simulink model "qr_array_cosim"  (R2017a)
settings: Solver=VariableStepAuto  StartTime=0.0  StopTime=600  RelTol=1e-3
values from neighbouring files (symbols this model uses):
  A = [0.69 0.5054 0.5914 0.5547 ... (first row only)    [load_data.m]
undefined symbols (not defined in the file or in its folder): N
libraries: xbsIndex_r4 x646, JTAGRuntimeCosim_r4 x1
(part 1 of 4)
settings Model: Creator=jhell  LastModifiedBy=jlh24

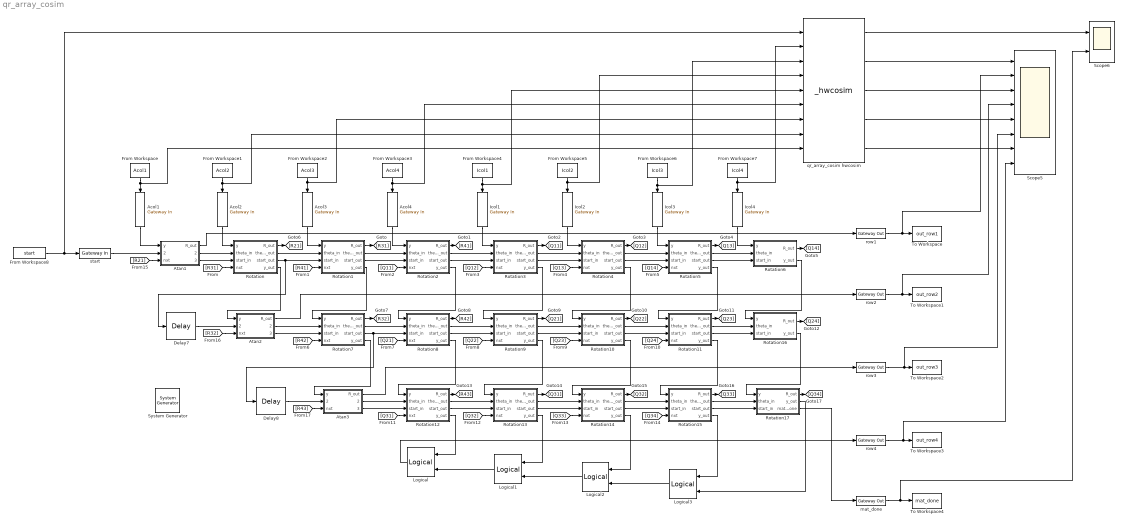
== system qr_array_cosim ==
  " System Generator" : xbsIndex_r4/ System Generator  Tag=genX  xilinxfamily=zynq  part=xc7z020  speed=-1  package=clg484  synthesis_tool=Vivado  clock_wrapper=Clock Enables  directory=./netlist_cosim  proj_type=Vivado  Synth_file=Vivado Synthesis Defaults  Impl_file=Vivado Implementation Defaults  testbench=off  simulink_period=1  sysclk_period=10  dcm_input_clock_period=10  incr_netlist=off  trim_vbits=Everywhere in SubSystem  dbl_ovrd=According to Block Masks  core_generation=According to Block Masks  run_coregen=off  deprecated_control=off  eval_field=0  block_type=sysgen
  Acol1 : xbsIndex_r4/Gateway In  gui_display_data_type=Fixed-point  arith_type="Signed  (2's comp)"  n_bits=16  bin_pt=13  preci_type=Single  exp_width=8  frac_width=24  rows=1  columns=1  quantization="Round  (unbiased: +/- Inf)"  overflow=Saturate  period=1  UseAsADC=off  ADCChannel='1'  interface=None  automatic_assignment=on  address_offset=hex2dec('00')  intf_name=''  intf_description=''  default_value=0  timing_constraint=None  locs_specified=off  LOCs={}  io_standard={}  inherit_from_input=off  hdl_port=on  dbl_ovrd=off  block_type=gatewayin
  Acol2 : xbsIndex_r4/Gateway In  gui_display_data_type=Fixed-point  arith_type="Signed  (2's comp)"  n_bits=16  bin_pt=13  preci_type=Single  exp_width=8  frac_width=24  rows=1  columns=1  quantization=Truncate  overflow=Saturate  period=1  UseAsADC=off  ADCChannel='1'  interface=None  automatic_assignment=on  address_offset=hex2dec('00')  intf_name=''  intf_description=''  default_value=0  timing_constraint=None  locs_specified=off  LOCs={}  io_standard={}  inherit_from_input=off  hdl_port=on  dbl_ovrd=off  block_type=gatewayin
  Acol3 : xbsIndex_r4/Gateway In  gui_display_data_type=Fixed-point  arith_type="Signed  (2's comp)"  n_bits=16  bin_pt=13  preci_type=Single  exp_width=8  frac_width=24  rows=1  columns=1  quantization=Truncate  overflow=Saturate  period=1  UseAsADC=off  ADCChannel='1'  interface=None  automatic_assignment=on  address_offset=hex2dec('00')  intf_name=''  intf_description=''  default_value=0  timing_constraint=None  locs_specified=off  LOCs={}  io_standard={}  inherit_from_input=off  hdl_port=on  dbl_ovrd=off  block_type=gatewayin
  Acol4 : xbsIndex_r4/Gateway In  gui_display_data_type=Fixed-point  arith_type="Signed  (2's comp)"  n_bits=16  bin_pt=13  preci_type=Single  exp_width=8  frac_width=24  rows=1  columns=1  quantization=Truncate  overflow=Saturate  period=1  UseAsADC=off  ADCChannel='1'  interface=None  automatic_assignment=on  address_offset=hex2dec('00')  intf_name=''  intf_description=''  default_value=0  timing_constraint=None  locs_specified=off  LOCs={}  io_standard={}  inherit_from_input=off  hdl_port=on  dbl_ovrd=off  block_type=gatewayin
  Atan1 : Subsystem
  Atan2 : Subsystem
  Atan3 : Subsystem
  Delay7 : xbsIndex_r4/Delay  rst=off  infoeditControl=Selection of Reset will increase slice count due to use of real FFs and instead of SRLs  en=off  latency=43  reg_retiming=off  dbl_ovrd=off  block_type=delay
  Delay8 : xbsIndex_r4/Delay  rst=off  infoeditControl=Selection of Reset will increase slice count due to use of real FFs and instead of SRLs  en=off  latency=43  reg_retiming=off  dbl_ovrd=off  block_type=delay
  From Workspace : FromWorkspace  VariableName=Acol1  SampleTime=0  Interpolate=off  OutputAfterFinalValue=Setting to zero
  From Workspace1 : FromWorkspace  VariableName=Acol2  SampleTime=0  Interpolate=off  OutputAfterFinalValue=Setting to zero
  From Workspace2 : FromWorkspace  VariableName=Acol3  SampleTime=0  Interpolate=off  OutputAfterFinalValue=Setting to zero
  From Workspace3 : FromWorkspace  VariableName=Acol4  SampleTime=0  Interpolate=off  OutputAfterFinalValue=Setting to zero
  From Workspace4 : FromWorkspace  VariableName=Icol1  SampleTime=0  Interpolate=off  OutputAfterFinalValue=Setting to zero
  From Workspace5 : FromWorkspace  VariableName=Icol2  SampleTime=0  Interpolate=off  OutputAfterFinalValue=Setting to zero
  From Workspace6 : FromWorkspace  VariableName=Icol3  SampleTime=0  Interpolate=off  OutputAfterFinalValue=Setting to zero
  From Workspace7 : FromWorkspace  VariableName=Icol4  SampleTime=0  Interpolate=off  OutputAfterFinalValue=Setting to zero
  From Workspace8 : FromWorkspace  VariableName=start  SampleTime=0
  Icol{1..4} (4 alike) : xbsIndex_r4/Gateway In  gui_display_data_type=Fixed-point  arith_type="Signed  (2's comp)"  n_bits=16  bin_pt=13  preci_type=Single  exp_width=8  frac_width=24  rows=1  columns=1  quantization=Truncate  overflow=Saturate  period=1  UseAsADC=off  ADCChannel='1'  interface=None  automatic_assignment=on  address_offset=hex2dec('00')  intf_name=''  intf_description=''  default_value=0  timing_constraint=None  locs_specified=off  LOCs={}  io_standard={}  inherit_from_input=off  hdl_port=on  dbl_ovrd=off  block_type=gatewayin
  Logical{,1..3} (4 alike) : xbsIndex_r4/Logical  logical_function=OR  inputs=2  en=off  latency=1  precision=Full  arith_type=Unsigned  n_bits=16  bin_pt=0  align_bp=on  dbl_ovrd=off  block_type=logical
  Rotation : Subsystem
  Rotation1 : Subsystem
  Rotation10 : Subsystem
  Rotation11 : Subsystem
  Rotation12 : Subsystem
  Rotation13 : Subsystem
  Rotation14 : Subsystem
  Rotation15 : Subsystem
  Rotation16 : Subsystem
  Rotation17 : Subsystem
  Rotation2 : Subsystem
  Rotation3 : Subsystem
  Rotation4 : Subsystem
  Rotation5 : Subsystem
  Rotation6 : Subsystem
  Rotation7 : Subsystem
  Rotation8 : Subsystem
  Rotation9 : Subsystem
  Scope5 : Scope  NumInputPorts=8
  Scope6 : Scope  NumInputPorts=2
  To Workspace : ToWorkspace  VariableName=out_row1  SampleTime=-1
  To Workspace1 : ToWorkspace  VariableName=out_row2  SampleTime=-1
  To Workspace2 : ToWorkspace  VariableName=out_row3  SampleTime=-1
  To Workspace3 : ToWorkspace  VariableName=out_row4  SampleTime=-1
  To Workspace4 : ToWorkspace  VariableName=mat_done  SampleTime=-1
  mat_done : xbsIndex_r4/Gateway Out  inherit_from_input=off  hdl_port=on  rows=1  columns=1  UseAsDAC=off  DACChannel='1'  interface=None  automatic_assignment=on  address_offset=hex2dec('00')  intf_name=''  intf_description=''  timing_constraint=None  locs_specified=off  LOCs={}  io_standard={}  block_type=gatewayout
  qr_array_cosim hwcosim : JTAGRuntimeCosim_r4/_hwcosim  clkSrc=Single Stepped  hasCombinationalPath=on  bitfileName=C:\ELEC522\hellar\Project_5\netlist_cosim\qr_array_cosim.bit  skipConfig=off  dispPartInfo=off  useZynqReconfigScript=on  cable=Auto Detect  speed=N/A  cablePort=N/A  cableLocation=Local  shareCable=off  design_xtable=|  engineDll=JTAGCosimEngine.dll  cableWaitTime=10  bscanPos=-1  IRLengths=[]  useWaitBox=1  hasBufgmux=on  Scheme=Cosim  useCmdProc=1  hasProc=0  useImpact=0  printLogFile=0  userChain=2  block_type=jtagcosim
      | {
      |     'clkWrapper' => 'qr_array_cosim',
      |     'burstMode' => false,
      |     'burstFifoDepth' => '1024',
      |     'shared_memories' => {},
      |     'clocksGcd' => 1,
      |     'device' => {
      |       'family' => 'zynq',
      |       'part' => 'xc7z020',
      |       'package' => 'clg484',
      |       'speed' => '-1',
      |     },
      |     'ports' => {
      |       'start' => {
      |         'direction' => 'in',
      |         'width' => 1,
      |         'name' => 'start',
      |         'period' => 1,
      |         'icon_text' => 'start',
      |         'type' => 'Bool',
      |         'arithmetic_type' => 'xlUnsigned',
      |         'dat_file' => 'qr_array_cosim_start.dat',
      |         'bin_pt' => 0,
      |         'addr_offset' => 0,
      |         'bd_port_index' => 0,
      |       },
      |       'icol4' => {
      |         'direction' => 'in',
      |         'width' => 16,
      |         'name' => 'icol4',
      |         'period' => 1,
      |         'icon_text' => 'Icol4',
      |         'type' => 'Fix_16_13',
      |         'arithmetic_type' => 'xlSigned',
      |         'dat_file' => 'qr_array_cosim_icol4.dat',
      |         'bin_pt' => 13,
      |         'addr_offset' => 4,
      |         'bd_port_index' => 1,
      |       },
      |       'icol3' => {
      |         'direction' => 'in',
      |         'width' => 16,
      |         'name' => 'icol3',
      |         'period' => 1,
      |         'icon_text' => 'Icol3',
      |         'type' => 'Fix_16_13',
      |         'arithmetic_type' => 'xlSigned',
      |         'dat_file' => 'qr_array_cosim_icol3.dat',
      |         'bin_pt' => 13,
      |         'addr_offset' => 8,
      |         'bd_port_index' => 2,
      |       },
      |       'icol2' => {
      |         'direction' => 'in',
      |         'width' => 16,
      |         'name' => 'icol2',
      |         'period' => 1,
      |         'icon_text' => 'Icol2',
      |         'type' => 'Fix_16_13',
      |         'arithmetic_type' => 'xlSigned',
      |         'dat_file' => 'qr_array_cosim_icol2.dat',
      |         'bin_pt' => 13,
      |         'addr_offset' => 12,
      |         'bd_port_index' => 3,
      |       },
      |       'icol1' => {
      |         'direction' => 'in',
      |         'width' => 16,
      |         'name' => 'icol1',
      |         'period' => 1,
      |         'icon_text' => 'Icol1',
      |         'type' => 'Fix_16_13',
      |         'arithmetic_type' => 'xlSigned',
      |         'dat_file' => 'qr_array_cosim_icol1.dat',
      |         'bin_pt' => 13,
      |         'addr_offset' => 16,
      |         'bd_port_index' => 4,
      |       },
      |       'acol4' => {
      |         'direction' => 'in',
      |         'width' => 16,
      |         'name' => 'acol4',
      |         'period' => 1,
      |         'icon_text' => 'Acol4',
      |         'type' => 'Fix_16_13',
      |         'arithmetic_type' => 'xlSigned',
      |         'dat_file' => 'qr_array_cosim_acol4.dat',
      |         'bin_pt' => 13,
      |         'addr_offset' => 20,
      |         'bd_port_index' => 5,
      |       },
      |       'acol3' => {
      |         'direction' => 'in',
      |         'width' => 16,
      |         'name' => 'acol3',
      |         'period' => 1,
      |         'icon_text' => 'Acol3',
      |         'type' => 'Fix_16_13',
      |         'arithmetic_type' => 'xlSigned',
      |         'dat_file' => 'qr_array_cosim_acol3.dat',
      |         'bin_pt' => 13,
      |         'addr_offset' => 24,
      |         'bd_port_index' => 6,
      |       },
      |       'acol2' => {
      |         'direction' => 'in',
      |         'width' => 16,
      |         'name' => 'acol2',
      |         'period' => 1,
      |         'icon_text' => 'Acol2',
      |         'type' => 'Fix_16_13',
      |         'arithmetic_type' => 'xlSigned',
      |         'dat_file' => 'qr_array_cosim_acol2.dat',
      |         'bin_pt' => 13,
      |         'addr_offset' => 28,
      |         'bd_port_index' => 7,
      |       },
      |       'acol1' => {
      |         'direction' => 'in',
      |         'width' => 16,
      |         'name' => 'acol1',
      |         'period' => 1,
      |         'icon_text' => 'Acol1',
      |         'type' => 'Fix_16_13',
      |         'arithmetic_type' => 'xlSigned',
      |         'dat_file' => 'qr_array_cosim_acol1.dat',
      |         'bin_pt' => 13,
      |         'addr_offset' => 32,
      |         'bd_port_index' => 8,
      |       },
      |       'mat_done' => {
      |         'direction' => 'out',
      |         'width' => 1,
      |         'name' => 'mat_done',
      |         'period' => 1,
      |         'icon_text' => 'mat_done',
      |         'type' => 'Bool',
      |         'arithmetic_type' => 'xlUnsigned',
      |         'dat_file' => 'qr_array_cosim_mat_done.dat',
      |         'bin_pt' => 0,
      |         'addr_offset' => 36,
      |         'bd_port_index' => 0,
      |       },
      |       'row1' => {
      |         'direction' => 'out',
      |         'width' => 16,
      |         'name' => 'row1',
      |         'period' => 1,
      |         'icon_text' => 'row1',
      |         'type' => 'Fix_16_13',
      |         'arithmetic_type' => 'xlSigned',
      |         'dat_file' => 'qr_array_cosim_row1.dat',
      |         'bin_pt' => 13,
      |         'addr_offset' => 40,
      |         'bd_port_index' => 1,
      |       },
      |       'row2' => {
      |         'direction' => 'out',
      |         'width' => 16,
      |         'name' => 'row2',
      |         'period' => 1,
      |         'icon_text' => 'row2',
      |         'type' => 'Fix_16_13',
      |         'arithmetic_type' => 'xlSigned',
      |         'dat_file' => 'qr_array_cosim_row2.dat',
      |         'bin_pt' => 13,
      |         'addr_offset' => 44,
      |         'bd_port_index' => 2,
      |       },
      |       'row3' => {
      |         'direction' => 'out',
      |         'width' => 16,
      |         'name' => 'row3',
      |         'period' => 1,
      |         'icon_text' => 'row3',
      |         'type' => 'Fix_16_13',
      |         'arithmetic_type' => 'xlSigned',
      |         'dat_file' => 'qr_array_cosim_row3.dat',
      |         'bin_pt' => 13,
      |         'addr_offset' => 48,
      |         'bd_port_index' => 3,
      |       },
      |       'row4' => {
      |         'direction' => 'out',
      |         'width' => 16,
      |         'name' => 'row4',
      |         'period' => 1,
      |         'icon_text' => 'row4',
      |         'type' => 'Fix_16_13',
      |         'arithmetic_type' => 'xlSigned',
      |         'dat_file' => 'qr_array_cosim_row4.dat',
      |         'bin_pt' => 13,
      |         'addr_offset' => 52,
      |         'bd_port_index' => 4,
      |       },
      |     },
      |   }
  row{1..4} (4 alike) : xbsIndex_r4/Gateway Out  inherit_from_input=off  hdl_port=on  rows=1  columns=1  UseAsDAC=off  DACChannel='1'  interface=None  automatic_assignment=on  address_offset=hex2dec('00')  intf_name=''  intf_description=''  timing_constraint=None  locs_specified=off  LOCs={}  io_standard={}  block_type=gatewayout
  start : xbsIndex_r4/Gateway In  gui_display_data_type=Boolean  arith_type=Boolean  n_bits=16  bin_pt=14  preci_type=Single  exp_width=8  frac_width=24  rows=1  columns=1  quantization="Round  (unbiased: +/- Inf)"  overflow=Saturate  period=1  UseAsADC=off  ADCChannel='1'  interface=None  automatic_assignment=on  address_offset=hex2dec('00')  intf_name=''  intf_description=''  default_value=0  timing_constraint=None  locs_specified=off  LOCs={}  io_standard={}  inherit_from_input=off  hdl_port=on  dbl_ovrd=off  block_type=gatewayin
  wires:
  From Workspace2/1 -> qr_array_cosim hwcosim/7, Acol3/1
  From Workspace3/1 -> qr_array_cosim hwcosim/6, Acol4/1
  From Workspace/1 -> qr_array_cosim hwcosim/9, Acol1/1
  From Workspace4/1 -> qr_array_cosim hwcosim/5, Icol1/1
  From Workspace5/1 -> qr_array_cosim hwcosim/4, Icol2/1
  From Workspace6/1 -> qr_array_cosim hwcosim/3, Icol3/1
  From Workspace7/1 -> qr_array_cosim hwcosim/2, Icol4/1
  Rotation/2(theta_out) -> Rotation1/2(theta_in)
  Rotation/3(start_out) -> Rotation1/3(start_in), Delay7/1
  Rotation1/2(theta_out) -> Rotation2/2(theta_in)
  Rotation1/3(start_out) -> Rotation2/3(start_in)
  Rotation2/2(theta_out) -> Rotation3/2(theta_in)
  Rotation2/3(start_out) -> Rotation3/3(start_in)
  Rotation3/2(theta_out) -> Rotation4/2(theta_in)
  Rotation3/3(start_out) -> Rotation4/3(start_in)
  Rotation4/2(theta_out) -> Rotation5/2(theta_in)
  Rotation4/3(start_out) -> Rotation5/3(start_in)
  Rotation5/2(theta_out) -> Rotation6/2(theta_in)
  Rotation5/3(start_out) -> Rotation6/3(start_in)
  Rotation1/1(R_out) -> [R31]
  [R31] -> Rotation/4(nxt)
  Rotation2/1(R_out) -> [R41]
  [R41] -> Rotation1/4(nxt)
  Rotation3/1(R_out) -> [Q11]
  Rotation4/1(R_out) -> [Q12]
  Rotation5/1(R_out) -> [Q13]
  Rotation6/1(R_out) -> [Q14]
  [Q11] -> Rotation2/4(nxt)
  [Q12] -> Rotation3/4(nxt)
  [Q13] -> Rotation4/4(nxt)
  [Q14] -> Rotation5/4(nxt)
  row1/1 -> Scope5/2, To Workspace/1
  Rotation7/2(theta_out) -> Rotation8/2(theta_in)
  Rotation7/3(start_out) -> Rotation8/3(start_in), Delay8/1
  Rotation8/2(theta_out) -> Rotation9/2(theta_in)
  Rotation8/3(start_out) -> Rotation9/3(start_in)
  Rotation9/2(theta_out) -> Rotation10/2(theta_in)
  Rotation9/3(start_out) -> Rotation10/3(start_in)
  Rotation10/2(theta_out) -> Rotation11/2(theta_in)
  Rotation10/3(start_out) -> Rotation11/3(start_in)
  Rotation1/4(y_out) -> Rotation7/1(y)
  Rotation2/4(y_out) -> Rotation8/1(y)
  Rotation3/4(y_out) -> Rotation9/1(y)
  Rotation4/4(y_out) -> Rotation10/1(y)
  Rotation5/4(y_out) -> Rotation11/1(y)
  Rotation11/3(start_out) -> Rotation16/3(start_in)
  Rotation11/2(theta_out) -> Rotation16/2(theta_in)
  Rotation6/2(y_out) -> Rotation16/1(y)
  Rotation16/2(y_out) -> Rotation17/1(y)
  Rotation/1(R_out) -> [R21]
  Rotation8/1(R_out) -> [R42]
  Rotation9/1(R_out) -> [Q21]
  Rotation10/1(R_out) -> [Q22]
  Rotation11/1(R_out) -> [Q23]
  Rotation16/1(R_out) -> [Q24]
  [R42] -> Rotation7/4(nxt)
  [Q21] -> Rotation8/4(nxt)
  [Q22] -> Rotation9/4(nxt)
  [Q23] -> Rotation10/4(nxt)
  [Q24] -> Rotation11/4(nxt)
  Rotation8/4(y_out) -> Rotation12/1(y)
  Rotation12/2(theta_out) -> Rotation13/2(theta_in)
  Rotation12/3(start_out) -> Rotation13/3(start_in)
  Rotation13/2(theta_out) -> Rotation14/2(theta_in)
  Rotation13/3(start_out) -> Rotation14/3(start_in)
  Rotation14/2(theta_out) -> Rotation15/2(theta_in)
  Rotation14/3(start_out) -> Rotation15/3(start_in)
  Rotation15/2(theta_out) -> Rotation17/2(theta_in)
  Rotation9/4(y_out) -> Rotation13/1(y)
  Rotation10/4(y_out) -> Rotation14/1(y)
  Rotation11/4(y_out) -> Rotation15/1(y)
  Rotation12/1(R_out) -> [R43]
  Rotation13/1(R_out) -> [Q31]
  Rotation14/1(R_out) -> [Q32]
  Rotation15/1(R_out) -> [Q33]
  Rotation17/1(R_out) -> [Q34]
  Rotation15/3(start_out) -> Rotation17/3(start_in)
  [Q31] -> Rotation12/4(nxt)
  [Q32] -> Rotation13/4(nxt)
  [Q33] -> Rotation14/4(nxt)
  [Q34] -> Rotation15/4(nxt)
  row2/1 -> Scope5/4, To Workspace1/1
  row3/1 -> Scope5/6, To Workspace2/1
  row4/1 -> Scope5/8, To Workspace3/1
  Atan1/2(theta_out) -> Rotation/2(theta_in)
  Atan1/3(start_out) -> Rotation/3(start_in)
  Atan1/1(R_out) -> row1/1
  [R21] -> Atan1/3(nxt)
  Acol1/1 -> Atan1/1(y)
  Atan2/2(theta_out) -> Rotation7/2(theta_in)
  Atan2/3(start_out) -> Rotation7/3(start_in)
  Atan2/1(R_out) -> row2/1
  Rotation/4(y_out) -> Atan2/1(y)
  [R32] -> Atan2/3(nxt)
  Atan3/3(start_out) -> Rotation12/3(start_in)
  Rotation7/4(y_out) -> Atan3/1(y)
  Atan3/1(R_out) -> row3/1
  From Workspace8/1 -> qr_array_cosim hwcosim/1, start/1
  start/1 -> Atan1/2(start_in)
  Acol2/1 -> Rotation/1(y)
  Acol3/1 -> Rotation1/1(y)
  Acol4/1 -> Rotation2/1(y)
  Icol1/1 -> Rotation3/1(y)
  Icol2/1 -> Rotation4/1(y)
  Icol3/1 -> Rotation5/1(y)
  Icol4/1 -> Rotation6/1(y)
  [R43] -> Atan3/3(nxt)
  Delay7/1 -> Atan2/2(start_in)
  Delay8/1 -> Atan3/2(start_in)
  Rotation7/1(R_out) -> [R32]
  Atan3/2(theta_out) -> Rotation12/2(theta_in)
  Rotation17/3(mat_done) -> mat_done/1
  mat_done/1 -> Scope6/2, To Workspace4/1
  Rotation12/4(y_out) -> Logical/1
  Logical1/1 -> Logical/2
  Rotation13/4(y_out) -> Logical1/1
  Rotation14/4(y_out) -> Logical2/1
  Logical2/1 -> Logical1/2
  Logical3/1 -> Logical2/2
  Rotation15/4(y_out) -> Logical3/1
  Rotation17/2(y_out) -> Logical3/2
  Logical/1 -> row4/1
  From Workspace1/1 -> qr_array_cosim hwcosim/8, Acol2/1
  qr_array_cosim hwcosim/2 -> Scope5/1
  qr_array_cosim hwcosim/3 -> Scope5/3
  qr_array_cosim hwcosim/4 -> Scope5/5
  qr_array_cosim hwcosim/5 -> Scope5/7
  qr_array_cosim hwcosim/1 -> Scope6/1

== system qr_array_cosim/Atan1 ==
  note: GenerateCordicEnable
  note: GenerateQRDone
  y : Inport
  start_in : Inport  Port=2
  nxt : Inport  Port=3
  Accumulator : xbsIndex_r4/Accumulator  operation=Add  n_bits=8  overflow=Wrap  scale=1  rst=on  hasbypass=off  infoeditControl=reset for floating point data type must be asserted for a minimum of 2 cycles  en=on  latency=1  msb_inp=100  msb=100  lsb=-100  use_behavioral_HDL=on  implementation=Fabric  dbl_ovrd=off  block_type=accum
  Constant : xbsIndex_r4/Constant  const=0  gui_display_data_type=Fixed-point  arith_type=Signed (2's comp)  n_bits=16  bin_pt=13  preci_type=Single  exp_width=8  frac_width=24  explicit_period=off  period=1  equ=P=C  opselect=C  inp2=PCIN>>17  opr=+  inp1=P  carry=CIN  dbl_ovrd=off  block_type=constant
  Constant1 : xbsIndex_r4/Constant  const=1  gui_display_data_type=Fixed-point  arith_type=Unsigned  n_bits=16  bin_pt=0  preci_type=Single  exp_width=8  frac_width=24  explicit_period=off  period=1  equ=P=C  opselect=C  inp2=PCIN>>17  opr=+  inp1=P  carry=CIN  dbl_ovrd=off  block_type=constant
  Constant2 : xbsIndex_r4/Constant  const=0  gui_display_data_type=Boolean  arith_type=Boolean  n_bits=16  bin_pt=14  preci_type=Single  exp_width=8  frac_width=24  explicit_period=off  period=1  equ=P=C  opselect=C  inp2=PCIN>>17  opr=+  inp1=P  carry=CIN  dbl_ovrd=off  block_type=constant
  Constant4 : xbsIndex_r4/Constant  const=0  gui_display_data_type=Fixed-point  arith_type=Signed (2's comp)  n_bits=16  bin_pt=13  preci_type=Single  exp_width=8  frac_width=24  explicit_period=off  period=1  equ=P=C  opselect=C  inp2=PCIN>>17  opr=+  inp1=P  carry=CIN  dbl_ovrd=off  block_type=constant
  Constant5 : xbsIndex_r4/Constant  const=0  gui_display_data_type=Fixed-point  arith_type=Unsigned  n_bits=16  bin_pt=0  preci_type=Single  exp_width=8  frac_width=24  explicit_period=off  period=1  equ=P=C  opselect=C  inp2=PCIN>>17  opr=+  inp1=P  carry=CIN  dbl_ovrd=off  block_type=constant
  Constant6 : xbsIndex_r4/Constant  const=4  gui_display_data_type=Fixed-point  arith_type=Unsigned  n_bits=16  bin_pt=0  preci_type=Single  exp_width=8  frac_width=24  explicit_period=off  period=1  equ=P=C  opselect=C  inp2=PCIN>>17  opr=+  inp1=P  carry=CIN  dbl_ovrd=off  block_type=constant
  Delay : xbsIndex_r4/Delay  rst=off  infoeditControl=Selection of Reset will increase slice count due to use of real FFs and instead of SRLs  en=off  latency=1  reg_retiming=off  dbl_ovrd=off  block_type=delay
  Delay4 : xbsIndex_r4/Delay  rst=off  infoeditControl=Selection of Reset will increase slice count due to use of real FFs and instead of SRLs  en=off  latency=4  reg_retiming=off  dbl_ovrd=off  block_type=delay
  Delay5 : xbsIndex_r4/Delay  rst=off  infoeditControl=Selection of Reset will increase slice count due to use of real FFs and instead of SRLs  en=off  latency=1  reg_retiming=off  dbl_ovrd=off  block_type=delay
  Delay6 : xbsIndex_r4/Delay  rst=off  infoeditControl=Selection of Reset will increase slice count due to use of real FFs and instead of SRLs  en=off  latency=44  reg_retiming=off  dbl_ovrd=off  block_type=delay
  Delay7 : xbsIndex_r4/Delay  rst=off  infoeditControl=Selection of Reset will increase slice count due to use of real FFs and instead of SRLs  en=off  latency=43  reg_retiming=off  dbl_ovrd=off  block_type=delay
  Delay8 : xbsIndex_r4/Delay  rst=off  infoeditControl=Selection of Reset will increase slice count due to use of real FFs and instead of SRLs  en=off  latency=2  reg_retiming=off  dbl_ovrd=off  block_type=delay
  Inverter : xbsIndex_r4/Inverter  en=off  latency=1  dbl_ovrd=off  block_type=inv
  Logical : xbsIndex_r4/Logical  logical_function=OR  inputs=2  en=off  latency=1  precision=Full  arith_type=Unsigned  n_bits=16  bin_pt=0  align_bp=on  dbl_ovrd=off  block_type=logical
  Logical3 : xbsIndex_r4/Logical  logical_function=XOR  inputs=2  en=off  latency=0  precision=Full  arith_type=Unsigned  n_bits=16  bin_pt=0  align_bp=on  dbl_ovrd=off  block_type=logical
  Logical4 : xbsIndex_r4/Logical  logical_function=OR  inputs=2  en=off  latency=1  precision=Full  arith_type=Unsigned  n_bits=16  bin_pt=0  align_bp=on  dbl_ovrd=off  block_type=logical
  Logical5 : xbsIndex_r4/Logical  logical_function=OR  inputs=2  en=off  latency=0  precision=Full  arith_type=Unsigned  n_bits=16  bin_pt=0  align_bp=on  dbl_ovrd=off  block_type=logical
  Logical6 : xbsIndex_r4/Logical  logical_function=XOR  inputs=2  en=off  latency=1  precision=Full  arith_type=Unsigned  n_bits=16  bin_pt=0  align_bp=on  dbl_ovrd=off  block_type=logical
  Logical7 : xbsIndex_r4/Logical  logical_function=OR  inputs=2  en=off  latency=1  precision=Full  arith_type=Unsigned  n_bits=16  bin_pt=0  align_bp=on  dbl_ovrd=off  block_type=logical
  Logical8 : xbsIndex_r4/Logical  logical_function=AND  inputs=2  en=off  latency=1  precision=Full  arith_type=Unsigned  n_bits=16  bin_pt=0  align_bp=on  dbl_ovrd=off  block_type=logical
  Mux{,1..3} (4 alike) : xbsIndex_r4/Mux  inputs=2  en=off  latency=1  precision=Full  arith_type=Unsigned  n_bits=16  bin_pt=14  quantization=Truncate  overflow=Wrap  dbl_ovrd=off  block_type=mux
  Register : xbsIndex_r4/Register  init=0  rst=on  en=on  dbl_ovrd=off  block_type=register
  Register2 : xbsIndex_r4/Register  init=0  rst=off  en=on  dbl_ovrd=off  block_type=register
  Relational : xbsIndex_r4/Relational  mode=a=b  op_type=Bool  en=off  latency=0  dbl_ovrd=off  block_type=relational
  Terminator{1..5} (5 alike) : Terminator
  Vivado HLS : xbsIndex_r4/Vivado HLS  anytable='C:/ELEC522/hellar/Project_4/cordic_revised/cordic_revised/solution1'  fast_sim=off  display_datatype=on  rate_propagation_method=Simulink system period  model_file_path=''  latency=1  block_type=hls
      settings: infoedit=This block allows including C,C++ and SystemC source files in System Generator for DSP designs.
  R_out : Outport
  theta_out : Outport  Port=2
  start_out : Outport  Port=3
  wires:
  Delay4/1 -> Vivado HLS/1
  Vivado HLS/2 -> Terminator2/1
  Constant4/1 -> Mux1/3
  Constant2/1 -> Vivado HLS/3
  Mux/1 -> Register/1
  Vivado HLS/1 -> Terminator4/1
  Constant/1 -> Vivado HLS/6
  y/1 -> Mux/3, Vivado HLS/4
  Vivado HLS/5 -> [R_vld]
  [R_out] -> Mux/2
  nxt/1 -> Mux2/2
  Vivado HLS/3 -> Terminator3/1
  Vivado HLS/6 -> Terminator5/1
  Vivado HLS/7 -> Terminator1/1
  Vivado HLS/8 -> Register2/1
  Vivado HLS/9 -> Register2/2
  start_in/1 -> [new_mat], Delay6/1
  Vivado HLS/4 -> [R_out]
  [done] -> Delay/1
  Delay/1 -> Register/2
  [R_vld] -> Delay8/1, Logical/2
  [reg_internal] -> Mux1/2
  Register/1 -> Mux2/3, [reg_internal]
  [done] -> Delay4/1
  [new_mat] -> Mux1/1
  [new_mat] -> Mux/1
  [new_mat] -> Logical/1
  [done] -> Mux2/1
  Logical/1 -> Register/3
  Delay8/1 -> [data_ready]
  Logical8/1 -> Vivado HLS/2, [enable]
  Register2/1 -> Inverter/1
  Delay6/1 -> start_out/1
  Mux2/1 -> R_out/1
  Relational/1 -> Logical4/2, Accumulator/2, [done]
  Mux1/1 -> Vivado HLS/5
  Inverter/1 -> theta_out/1
  Delay5/1 -> Logical3/1, Accumulator/3
  Logical3/1 -> Delay5/1
  Logical4/1 -> Logical3/2
  [new_mat] -> Logical4/1
  Constant6/1 -> Relational/2
  Constant5/1 -> Mux3/2
  Constant1/1 -> Mux3/3
  Accumulator/1 -> Relational/1
  Mux3/1 -> Accumulator/1
  [enable] -> Mux3/1
  Logical5/1 -> Logical8/1
  Logical7/1 -> Logical6/2
  Logical6/1 -> Logical6/1, Logical8/2
  [done] -> Logical7/2
  [new_mat] -> Delay7/1, Logical7/1
  Delay7/1 -> Logical5/2
  [data_ready] -> Logical5/1

== system qr_array_cosim/Atan2 ==
  note: GenerateCordicEnable
  note: GenerateQRDone
  y : Inport
  start_in : Inport  Port=2
  nxt : Inport  Port=3
  Accumulator : xbsIndex_r4/Accumulator  operation=Add  n_bits=8  overflow=Wrap  scale=1  rst=on  hasbypass=off  infoeditControl=reset for floating point data type must be asserted for a minimum of 2 cycles  en=on  latency=1  msb_inp=100  msb=100  lsb=-100  use_behavioral_HDL=on  implementation=Fabric  dbl_ovrd=off  block_type=accum
  Constant : xbsIndex_r4/Constant  const=0  gui_display_data_type=Fixed-point  arith_type=Signed (2's comp)  n_bits=16  bin_pt=13  preci_type=Single  exp_width=8  frac_width=24  explicit_period=off  period=1  equ=P=C  opselect=C  inp2=PCIN>>17  opr=+  inp1=P  carry=CIN  dbl_ovrd=off  block_type=constant
  Constant1 : xbsIndex_r4/Constant  const=1  gui_display_data_type=Fixed-point  arith_type=Unsigned  n_bits=16  bin_pt=0  preci_type=Single  exp_width=8  frac_width=24  explicit_period=off  period=1  equ=P=C  opselect=C  inp2=PCIN>>17  opr=+  inp1=P  carry=CIN  dbl_ovrd=off  block_type=constant
  Constant2 : xbsIndex_r4/Constant  const=0  gui_display_data_type=Boolean  arith_type=Boolean  n_bits=16  bin_pt=14  preci_type=Single  exp_width=8  frac_width=24  explicit_period=off  period=1  equ=P=C  opselect=C  inp2=PCIN>>17  opr=+  inp1=P  carry=CIN  dbl_ovrd=off  block_type=constant
  Constant4 : xbsIndex_r4/Constant  const=0  gui_display_data_type=Fixed-point  arith_type=Signed (2's comp)  n_bits=16  bin_pt=13  preci_type=Single  exp_width=8  frac_width=24  explicit_period=off  period=1  equ=P=C  opselect=C  inp2=PCIN>>17  opr=+  inp1=P  carry=CIN  dbl_ovrd=off  block_type=constant
  Constant5 : xbsIndex_r4/Constant  const=0  gui_display_data_type=Fixed-point  arith_type=Unsigned  n_bits=16  bin_pt=0  preci_type=Single  exp_width=8  frac_width=24  explicit_period=off  period=1  equ=P=C  opselect=C  inp2=PCIN>>17  opr=+  inp1=P  carry=CIN  dbl_ovrd=off  block_type=constant
  Constant6 : xbsIndex_r4/Constant  const=3  gui_display_data_type=Fixed-point  arith_type=Unsigned  n_bits=16  bin_pt=0  preci_type=Single  exp_width=8  frac_width=24  explicit_period=off  period=1  equ=P=C  opselect=C  inp2=PCIN>>17  opr=+  inp1=P  carry=CIN  dbl_ovrd=off  block_type=constant
  Delay : xbsIndex_r4/Delay  rst=off  infoeditControl=Selection of Reset will increase slice count due to use of real FFs and instead of SRLs  en=off  latency=1  reg_retiming=off  dbl_ovrd=off  block_type=delay
  Delay4 : xbsIndex_r4/Delay  rst=off  infoeditControl=Selection of Reset will increase slice count due to use of real FFs and instead of SRLs  en=off  latency=4  reg_retiming=off  dbl_ovrd=off  block_type=delay
  Delay5 : xbsIndex_r4/Delay  rst=off  infoeditControl=Selection of Reset will increase slice count due to use of real FFs and instead of SRLs  en=off  latency=1  reg_retiming=off  dbl_ovrd=off  block_type=delay
  Delay6 : xbsIndex_r4/Delay  rst=off  infoeditControl=Selection of Reset will increase slice count due to use of real FFs and instead of SRLs  en=off  latency=44  reg_retiming=off  dbl_ovrd=off  block_type=delay
  Delay7 : xbsIndex_r4/Delay  rst=off  infoeditControl=Selection of Reset will increase slice count due to use of real FFs and instead of SRLs  en=off  latency=43  reg_retiming=off  dbl_ovrd=off  block_type=delay
  Delay8 : xbsIndex_r4/Delay  rst=off  infoeditControl=Selection of Reset will increase slice count due to use of real FFs and instead of SRLs  en=off  latency=2  reg_retiming=off  dbl_ovrd=off  block_type=delay
  Inverter : xbsIndex_r4/Inverter  en=off  latency=1  dbl_ovrd=off  block_type=inv
  Logical : xbsIndex_r4/Logical  logical_function=OR  inputs=2  en=off  latency=1  precision=Full  arith_type=Unsigned  n_bits=16  bin_pt=0  align_bp=on  dbl_ovrd=off  block_type=logical
  Logical3 : xbsIndex_r4/Logical  logical_function=XOR  inputs=2  en=off  latency=0  precision=Full  arith_type=Unsigned  n_bits=16  bin_pt=0  align_bp=on  dbl_ovrd=off  block_type=logical
  Logical4 : xbsIndex_r4/Logical  logical_function=OR  inputs=2  en=off  latency=1  precision=Full  arith_type=Unsigned  n_bits=16  bin_pt=0  align_bp=on  dbl_ovrd=off  block_type=logical
  Logical5 : xbsIndex_r4/Logical  logical_function=OR  inputs=2  en=off  latency=0  precision=Full  arith_type=Unsigned  n_bits=16  bin_pt=0  align_bp=on  dbl_ovrd=off  block_type=logical
  Logical6 : xbsIndex_r4/Logical  logical_function=XOR  inputs=2  en=off  latency=1  precision=Full  arith_type=Unsigned  n_bits=16  bin_pt=0  align_bp=on  dbl_ovrd=off  block_type=logical
  Logical7 : xbsIndex_r4/Logical  logical_function=OR  inputs=2  en=off  latency=1  precision=Full  arith_type=Unsigned  n_bits=16  bin_pt=0  align_bp=on  dbl_ovrd=off  block_type=logical
  Logical8 : xbsIndex_r4/Logical  logical_function=AND  inputs=2  en=off  latency=1  precision=Full  arith_type=Unsigned  n_bits=16  bin_pt=0  align_bp=on  dbl_ovrd=off  block_type=logical
  Mux{,1..3} (4 alike) : xbsIndex_r4/Mux  inputs=2  en=off  latency=1  precision=Full  arith_type=Unsigned  n_bits=16  bin_pt=14  quantization=Truncate  overflow=Wrap  dbl_ovrd=off  block_type=mux
  Register : xbsIndex_r4/Register  init=0  rst=on  en=on  dbl_ovrd=off  block_type=register
  Register2 : xbsIndex_r4/Register  init=0  rst=off  en=on  dbl_ovrd=off  block_type=register
  Relational : xbsIndex_r4/Relational  mode=a=b  op_type=Bool  en=off  latency=0  dbl_ovrd=off  block_type=relational
  Terminator{1..5} (5 alike) : Terminator
  Vivado HLS : xbsIndex_r4/Vivado HLS  anytable='C:/ELEC522/hellar/Project_4/cordic_revised/cordic_revised/solution1'  fast_sim=off  display_datatype=on  rate_propagation_method=Simulink system period  model_file_path=''  latency=1  block_type=hls
      settings: infoedit=This block allows including C,C++ and SystemC source files in System Generator for DSP designs.
  R_out : Outport
  theta_out : Outport  Port=2
  start_out : Outport  Port=3
  wires:
  Delay4/1 -> Vivado HLS/1
  Vivado HLS/2 -> Terminator2/1
  Constant4/1 -> Mux1/3
  Constant2/1 -> Vivado HLS/3
  Mux/1 -> Register/1
  Vivado HLS/1 -> Terminator4/1
  Constant/1 -> Vivado HLS/6
  y/1 -> Mux/3, Vivado HLS/4
  Vivado HLS/5 -> [R_vld]
  [R_out] -> Mux/2
  nxt/1 -> Mux2/2
  Vivado HLS/3 -> Terminator3/1
  Vivado HLS/6 -> Terminator5/1
  Vivado HLS/7 -> Terminator1/1
  Vivado HLS/8 -> Register2/1
  Vivado HLS/9 -> Register2/2
  start_in/1 -> [new_mat], Delay6/1
  Vivado HLS/4 -> [R_out]
  [done] -> Delay/1
  Delay/1 -> Register/2
  [R_vld] -> Delay8/1, Logical/2
  [reg_internal] -> Mux1/2
  Register/1 -> Mux2/3, [reg_internal]
  [done] -> Delay4/1
  [new_mat] -> Mux1/1
  [new_mat] -> Mux/1
  [new_mat] -> Logical/1
  [done] -> Mux2/1
  Logical/1 -> Register/3
  Delay8/1 -> [data_ready]
  Logical8/1 -> Vivado HLS/2, [enable]
  Register2/1 -> Inverter/1
  Delay6/1 -> start_out/1
  Mux2/1 -> R_out/1
  Relational/1 -> Logical4/2, Accumulator/2, [done]
  Mux1/1 -> Vivado HLS/5
  Inverter/1 -> theta_out/1
  Delay5/1 -> Logical3/1, Accumulator/3
  Logical3/1 -> Delay5/1
  Logical4/1 -> Logical3/2
  [new_mat] -> Logical4/1
  Constant6/1 -> Relational/2
  Constant5/1 -> Mux3/2
  Constant1/1 -> Mux3/3
  Accumulator/1 -> Relational/1
  Mux3/1 -> Accumulator/1
  [enable] -> Mux3/1
  Logical5/1 -> Logical8/1
  Logical7/1 -> Logical6/2
  Logical6/1 -> Logical6/1, Logical8/2
  [done] -> Logical7/2
  [new_mat] -> Delay7/1, Logical7/1
  Delay7/1 -> Logical5/2
  [data_ready] -> Logical5/1

== system qr_array_cosim/Atan3 ==
  note: GenerateCordicEnable
  note: GenerateQRDone
  y : Inport
  start_in : Inport  Port=2
  nxt : Inport  Port=3
  Accumulator : xbsIndex_r4/Accumulator  operation=Add  n_bits=8  overflow=Wrap  scale=1  rst=on  hasbypass=off  infoeditControl=reset for floating point data type must be asserted for a minimum of 2 cycles  en=on  latency=1  msb_inp=100  msb=100  lsb=-100  use_behavioral_HDL=on  implementation=Fabric  dbl_ovrd=off  block_type=accum
  Constant : xbsIndex_r4/Constant  const=0  gui_display_data_type=Fixed-point  arith_type=Signed (2's comp)  n_bits=16  bin_pt=13  preci_type=Single  exp_width=8  frac_width=24  explicit_period=off  period=1  equ=P=C  opselect=C  inp2=PCIN>>17  opr=+  inp1=P  carry=CIN  dbl_ovrd=off  block_type=constant
  Constant1 : xbsIndex_r4/Constant  const=1  gui_display_data_type=Fixed-point  arith_type=Unsigned  n_bits=16  bin_pt=0  preci_type=Single  exp_width=8  frac_width=24  explicit_period=off  period=1  equ=P=C  opselect=C  inp2=PCIN>>17  opr=+  inp1=P  carry=CIN  dbl_ovrd=off  block_type=constant
  Constant2 : xbsIndex_r4/Constant  const=0  gui_display_data_type=Boolean  arith_type=Boolean  n_bits=16  bin_pt=14  preci_type=Single  exp_width=8  frac_width=24  explicit_period=off  period=1  equ=P=C  opselect=C  inp2=PCIN>>17  opr=+  inp1=P  carry=CIN  dbl_ovrd=off  block_type=constant
  Constant4 : xbsIndex_r4/Constant  const=0  gui_display_data_type=Fixed-point  arith_type=Signed (2's comp)  n_bits=16  bin_pt=13  preci_type=Single  exp_width=8  frac_width=24  explicit_period=off  period=1  equ=P=C  opselect=C  inp2=PCIN>>17  opr=+  inp1=P  carry=CIN  dbl_ovrd=off  block_type=constant
  Constant5 : xbsIndex_r4/Constant  const=0  gui_display_data_type=Fixed-point  arith_type=Unsigned  n_bits=16  bin_pt=0  preci_type=Single  exp_width=8  frac_width=24  explicit_period=off  period=1  equ=P=C  opselect=C  inp2=PCIN>>17  opr=+  inp1=P  carry=CIN  dbl_ovrd=off  block_type=constant
  Constant6 : xbsIndex_r4/Constant  const=2  gui_display_data_type=Fixed-point  arith_type=Unsigned  n_bits=16  bin_pt=0  preci_type=Single  exp_width=8  frac_width=24  explicit_period=off  period=1  equ=P=C  opselect=C  inp2=PCIN>>17  opr=+  inp1=P  carry=CIN  dbl_ovrd=off  block_type=constant
  Delay : xbsIndex_r4/Delay  rst=off  infoeditControl=Selection of Reset will increase slice count due to use of real FFs and instead of SRLs  en=off  latency=1  reg_retiming=off  dbl_ovrd=off  block_type=delay
  Delay4 : xbsIndex_r4/Delay  rst=off  infoeditControl=Selection of Reset will increase slice count due to use of real FFs and instead of SRLs  en=off  latency=4  reg_retiming=off  dbl_ovrd=off  block_type=delay
  Delay5 : xbsIndex_r4/Delay  rst=off  infoeditControl=Selection of Reset will increase slice count due to use of real FFs and instead of SRLs  en=off  latency=1  reg_retiming=off  dbl_ovrd=off  block_type=delay
  Delay6 : xbsIndex_r4/Delay  rst=off  infoeditControl=Selection of Reset will increase slice count due to use of real FFs and instead of SRLs  en=off  latency=44  reg_retiming=off  dbl_ovrd=off  block_type=delay
  Delay7 : xbsIndex_r4/Delay  rst=off  infoeditControl=Selection of Reset will increase slice count due to use of real FFs and instead of SRLs  en=off  latency=43  reg_retiming=off  dbl_ovrd=off  block_type=delay
  Delay8 : xbsIndex_r4/Delay  rst=off  infoeditControl=Selection of Reset will increase slice count due to use of real FFs and instead of SRLs  en=off  latency=2  reg_retiming=off  dbl_ovrd=off  block_type=delay
  Inverter : xbsIndex_r4/Inverter  en=off  latency=1  dbl_ovrd=off  block_type=inv
  Logical : xbsIndex_r4/Logical  logical_function=OR  inputs=2  en=off  latency=1  precision=Full  arith_type=Unsigned  n_bits=16  bin_pt=0  align_bp=on  dbl_ovrd=off  block_type=logical
  Logical3 : xbsIndex_r4/Logical  logical_function=XOR  inputs=2  en=off  latency=0  precision=Full  arith_type=Unsigned  n_bits=16  bin_pt=0  align_bp=on  dbl_ovrd=off  block_type=logical
  Logical4 : xbsIndex_r4/Logical  logical_function=OR  inputs=2  en=off  latency=1  precision=Full  arith_type=Unsigned  n_bits=16  bin_pt=0  align_bp=on  dbl_ovrd=off  block_type=logical
  Logical5 : xbsIndex_r4/Logical  logical_function=OR  inputs=2  en=off  latency=0  precision=Full  arith_type=Unsigned  n_bits=16  bin_pt=0  align_bp=on  dbl_ovrd=off  block_type=logical
  Logical6 : xbsIndex_r4/Logical  logical_function=XOR  inputs=2  en=off  latency=1  precision=Full  arith_type=Unsigned  n_bits=16  bin_pt=0  align_bp=on  dbl_ovrd=off  block_type=logical
  Logical7 : xbsIndex_r4/Logical  logical_function=OR  inputs=2  en=off  latency=1  precision=Full  arith_type=Unsigned  n_bits=16  bin_pt=0  align_bp=on  dbl_ovrd=off  block_type=logical
  Logical8 : xbsIndex_r4/Logical  logical_function=AND  inputs=2  en=off  latency=1  precision=Full  arith_type=Unsigned  n_bits=16  bin_pt=0  align_bp=on  dbl_ovrd=off  block_type=logical
  Mux{,1..3} (4 alike) : xbsIndex_r4/Mux  inputs=2  en=off  latency=1  precision=Full  arith_type=Unsigned  n_bits=16  bin_pt=14  quantization=Truncate  overflow=Wrap  dbl_ovrd=off  block_type=mux
  Register : xbsIndex_r4/Register  init=0  rst=on  en=on  dbl_ovrd=off  block_type=register
  Register2 : xbsIndex_r4/Register  init=0  rst=off  en=on  dbl_ovrd=off  block_type=register
  Relational : xbsIndex_r4/Relational  mode=a=b  op_type=Bool  en=off  latency=0  dbl_ovrd=off  block_type=relational
  Terminator{1..5} (5 alike) : Terminator
  Vivado HLS : xbsIndex_r4/Vivado HLS  anytable='C:/ELEC522/hellar/Project_4/cordic_revised/cordic_revised/solution1'  fast_sim=off  display_datatype=on  rate_propagation_method=Simulink system period  model_file_path=''  latency=1  block_type=hls
      settings: infoedit=This block allows including C,C++ and SystemC source files in System Generator for DSP designs.
  R_out : Outport
  theta_out : Outport  Port=2
  start_out : Outport  Port=3
  wires:
  Delay4/1 -> Vivado HLS/1
  Vivado HLS/2 -> Terminator2/1
  Constant4/1 -> Mux1/3
  Constant2/1 -> Vivado HLS/3
  Mux/1 -> Register/1
  Vivado HLS/1 -> Terminator4/1
  Constant/1 -> Vivado HLS/6
  y/1 -> Mux/3, Vivado HLS/4
  Vivado HLS/5 -> [R_vld]
  [R_out] -> Mux/2
  nxt/1 -> Mux2/2
  Vivado HLS/3 -> Terminator3/1
  Vivado HLS/6 -> Terminator5/1
  Vivado HLS/7 -> Terminator1/1
  Vivado HLS/8 -> Register2/1
  Vivado HLS/9 -> Register2/2
  start_in/1 -> [new_mat], Delay6/1
  Vivado HLS/4 -> [R_out]
  [done] -> Delay/1
  Delay/1 -> Register/2
  [R_vld] -> Delay8/1, Logical/2
  [reg_internal] -> Mux1/2
  Register/1 -> Mux2/3, [reg_internal]
  [done] -> Delay4/1
  [new_mat] -> Mux1/1
  [new_mat] -> Mux/1
  [new_mat] -> Logical/1
  [done] -> Mux2/1
  Logical/1 -> Register/3
  Delay8/1 -> [data_ready]
  Logical8/1 -> Vivado HLS/2, [enable]
  Register2/1 -> Inverter/1
  Delay6/1 -> start_out/1
  Mux2/1 -> R_out/1
  Relational/1 -> Logical4/2, Accumulator/2, [done]
  Mux1/1 -> Vivado HLS/5
  Inverter/1 -> theta_out/1
  Delay5/1 -> Logical3/1, Accumulator/3
  Logical3/1 -> Delay5/1
  Logical4/1 -> Logical3/2
  [new_mat] -> Logical4/1
  Constant6/1 -> Relational/2
  Constant5/1 -> Mux3/2
  Constant1/1 -> Mux3/3
  Accumulator/1 -> Relational/1
  Mux3/1 -> Accumulator/1
  [enable] -> Mux3/1
  Logical5/1 -> Logical8/1
  Logical7/1 -> Logical6/2
  Logical6/1 -> Logical6/1, Logical8/2
  [done] -> Logical7/2
  [new_mat] -> Delay7/1, Logical7/1
  Delay7/1 -> Logical5/2
  [data_ready] -> Logical5/1

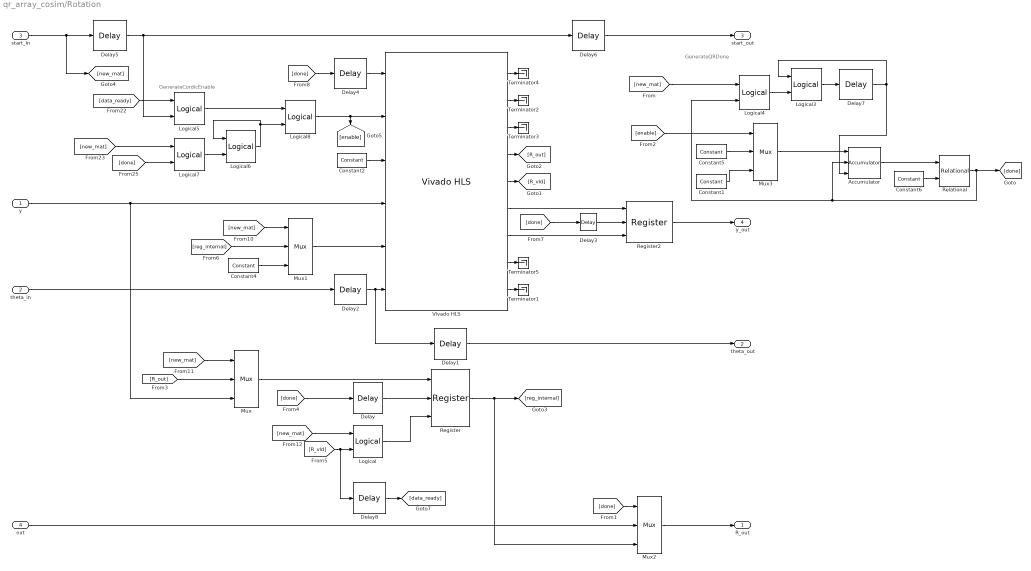
== system qr_array_cosim/Rotation ==
  note: GenerateQRDone
  note: GenerateCordicEnable
  y : Inport
  theta_in : Inport  Port=2
  start_in : Inport  Port=3
  nxt : Inport  Port=4
  Accumulator : xbsIndex_r4/Accumulator  operation=Add  n_bits=8  overflow=Wrap  scale=1  rst=on  hasbypass=off  infoeditControl=reset for floating point data type must be asserted for a minimum of 2 cycles  en=on  latency=1  msb_inp=100  msb=100  lsb=-100  use_behavioral_HDL=on  implementation=Fabric  dbl_ovrd=off  block_type=accum
  Constant1 : xbsIndex_r4/Constant  const=1  gui_display_data_type=Fixed-point  arith_type=Unsigned  n_bits=16  bin_pt=0  preci_type=Single  exp_width=8  frac_width=24  explicit_period=off  period=1  equ=P=C  opselect=C  inp2=PCIN>>17  opr=+  inp1=P  carry=CIN  dbl_ovrd=off  block_type=constant
  Constant2 : xbsIndex_r4/Constant  const=1  gui_display_data_type=Boolean  arith_type=Boolean  n_bits=16  bin_pt=14  preci_type=Single  exp_width=8  frac_width=24  explicit_period=off  period=1  equ=P=C  opselect=C  inp2=PCIN>>17  opr=+  inp1=P  carry=CIN  dbl_ovrd=off  block_type=constant
  Constant4 : xbsIndex_r4/Constant  const=0  gui_display_data_type=Fixed-point  arith_type=Signed (2's comp)  n_bits=16  bin_pt=13  preci_type=Single  exp_width=8  frac_width=24  explicit_period=off  period=1  equ=P=C  opselect=C  inp2=PCIN>>17  opr=+  inp1=P  carry=CIN  dbl_ovrd=off  block_type=constant
  Constant5 : xbsIndex_r4/Constant  const=0  gui_display_data_type=Fixed-point  arith_type=Unsigned  n_bits=16  bin_pt=0  preci_type=Single  exp_width=8  frac_width=24  explicit_period=off  period=1  equ=P=C  opselect=C  inp2=PCIN>>17  opr=+  inp1=P  carry=CIN  dbl_ovrd=off  block_type=constant
  Constant6 : xbsIndex_r4/Constant  const=4  gui_display_data_type=Fixed-point  arith_type=Unsigned  n_bits=16  bin_pt=0  preci_type=Single  exp_width=8  frac_width=24  explicit_period=off  period=1  equ=P=C  opselect=C  inp2=PCIN>>17  opr=+  inp1=P  carry=CIN  dbl_ovrd=off  block_type=constant
  Delay{,3,6..7} (4 alike) : xbsIndex_r4/Delay  rst=off  infoeditControl=Selection of Reset will increase slice count due to use of real FFs and instead of SRLs  en=off  latency=1  reg_retiming=off  dbl_ovrd=off  block_type=delay
  Delay1 : xbsIndex_r4/Delay  rst=off  infoeditControl=Selection of Reset will increase slice count due to use of real FFs and instead of SRLs  en=off  latency=41  reg_retiming=off  dbl_ovrd=off  block_type=delay
  Delay2 : xbsIndex_r4/Delay  rst=off  infoeditControl=Selection of Reset will increase slice count due to use of real FFs and instead of SRLs  en=off  latency=2  reg_retiming=off  dbl_ovrd=off  block_type=delay
  Delay4 : xbsIndex_r4/Delay  rst=off  infoeditControl=Selection of Reset will increase slice count due to use of real FFs and instead of SRLs  en=off  latency=4  reg_retiming=off  dbl_ovrd=off  block_type=delay
  Delay5 : xbsIndex_r4/Delay  rst=off  infoeditControl=Selection of Reset will increase slice count due to use of real FFs and instead of SRLs  en=off  latency=43  reg_retiming=off  dbl_ovrd=off  block_type=delay
  Delay8 : xbsIndex_r4/Delay  rst=off  infoeditControl=Selection of Reset will increase slice count due to use of real FFs and instead of SRLs  en=off  latency=2  reg_retiming=off  dbl_ovrd=off  block_type=delay
  Logical : xbsIndex_r4/Logical  logical_function=OR  inputs=2  en=off  latency=1  precision=Full  arith_type=Unsigned  n_bits=16  bin_pt=0  align_bp=on  dbl_ovrd=off  block_type=logical
  Logical3 : xbsIndex_r4/Logical  logical_function=XOR  inputs=2  en=off  latency=0  precision=Full  arith_type=Unsigned  n_bits=16  bin_pt=0  align_bp=on  dbl_ovrd=off  block_type=logical
  Logical4 : xbsIndex_r4/Logical  logical_function=OR  inputs=2  en=off  latency=1  precision=Full  arith_type=Unsigned  n_bits=16  bin_pt=0  align_bp=on  dbl_ovrd=off  block_type=logical
  Logical5 : xbsIndex_r4/Logical  logical_function=OR  inputs=2  en=off  latency=0  precision=Full  arith_type=Unsigned  n_bits=16  bin_pt=0  align_bp=on  dbl_ovrd=off  block_type=logical
  Logical6 : xbsIndex_r4/Logical  logical_function=XOR  inputs=2  en=off  latency=1  precision=Full  arith_type=Unsigned  n_bits=16  bin_pt=0  align_bp=on  dbl_ovrd=off  block_type=logical
  Logical7 : xbsIndex_r4/Logical  logical_function=OR  inputs=2  en=off  latency=1  precision=Full  arith_type=Unsigned  n_bits=16  bin_pt=0  align_bp=on  dbl_ovrd=off  block_type=logical
  Logical8 : xbsIndex_r4/Logical  logical_function=AND  inputs=2  en=off  latency=1  precision=Full  arith_type=Unsigned  n_bits=16  bin_pt=0  align_bp=on  dbl_ovrd=off  block_type=logical
  Mux{,1..3} (4 alike) : xbsIndex_r4/Mux  inputs=2  en=off  latency=1  precision=Full  arith_type=Unsigned  n_bits=16  bin_pt=14  quantization=Truncate  overflow=Wrap  dbl_ovrd=off  block_type=mux
  Register : xbsIndex_r4/Register  init=0  rst=on  en=on  dbl_ovrd=off  block_type=register
  Register2 : xbsIndex_r4/Register  init=0  rst=on  en=on  dbl_ovrd=off  block_type=register
  Relational : xbsIndex_r4/Relational  mode=a=b  op_type=Bool  en=off  latency=0  dbl_ovrd=off  block_type=relational
  Terminator{1..5} (5 alike) : Terminator
  Vivado HLS : xbsIndex_r4/Vivado HLS  anytable='C:/ELEC522/hellar/Project_4/cordic_revised/cordic_revised/solution1'  fast_sim=off  display_datatype=on  rate_propagation_method=Simulink system period  model_file_path=''  latency=1  block_type=hls
      settings: infoedit=This block allows including C,C++ and SystemC source files in System Generator for DSP designs.
  R_out : Outport
  theta_out : Outport  Port=2
  start_out : Outport  Port=3
  y_out : Outport  Port=4
  wires:
  [done] -> Delay3/1
  Delay8/1 -> [data_ready]
  [R_vld] -> Delay8/1, Logical/2
  [done] -> Mux2/1
  [new_mat] -> Mux/1
  [done] -> Delay4/1
  [new_mat] -> Mux1/1
  [reg_internal] -> Mux1/2
  Delay4/1 -> Vivado HLS/1
  Logical/1 -> Register/3
  [done] -> Delay/1
  [new_mat] -> Logical/1
  theta_in/1 -> Delay2/1
  Register/1 -> Mux2/3, [reg_internal]
  Delay6/1 -> start_out/1
  Mux/1 -> Register/1
  Vivado HLS/3 -> Terminator3/1
  Vivado HLS/5 -> [R_vld]
  [R_out] -> Mux/2
  Delay/1 -> Register/2
  y/1 -> Vivado HLS/4, Mux/3
  Vivado HLS/1 -> Terminator4/1
  Vivado HLS/4 -> [R_out]
  Mux2/1 -> R_out/1
  Constant4/1 -> Mux1/3
  start_in/1 -> [new_mat], Delay5/1
  nxt/1 -> Mux2/2
  Vivado HLS/2 -> Terminator2/1
  Constant2/1 -> Vivado HLS/3
  Logical8/1 -> Vivado HLS/2, [enable]
  Relational/1 -> Logical4/2, Accumulator/2, [done]
  Vivado HLS/8 -> Terminator5/1
  Vivado HLS/9 -> Terminator1/1
  Vivado HLS/6 -> Register2/1
  Vivado HLS/7 -> Register2/3
  Delay1/1 -> theta_out/1
  Delay2/1 -> Delay1/1, Vivado HLS/6
  Mux1/1 -> Vivado HLS/5
  Delay3/1 -> Register2/2
  Register2/1 -> y_out/1
  Logical5/1 -> Logical8/1
  Logical7/1 -> Logical6/2
  Logical6/1 -> Logical6/1, Logical8/2
  [done] -> Logical7/2
  [new_mat] -> Logical7/1
  [data_ready] -> Logical5/1
  Delay5/1 -> Delay6/1, Logical5/2
  Delay7/1 -> Logical3/1, Accumulator/3
  Logical3/1 -> Delay7/1
  Logical4/1 -> Logical3/2
  [new_mat] -> Logical4/1
  Constant6/1 -> Relational/2
  Constant5/1 -> Mux3/2
  Constant1/1 -> Mux3/3
  Accumulator/1 -> Relational/1
  Mux3/1 -> Accumulator/1
  [enable] -> Mux3/1
